simulink library "slib_spectrum_analyser"  (R2020a)
settings: Solver=VariableStepAuto  StartTime=0.0  StopTime=10.0  RelTol=1e-3
libraries: hdlsllib x104, simulink x55, dsphdlxfrm x11, $bdroot x5
(part 2 of 3)

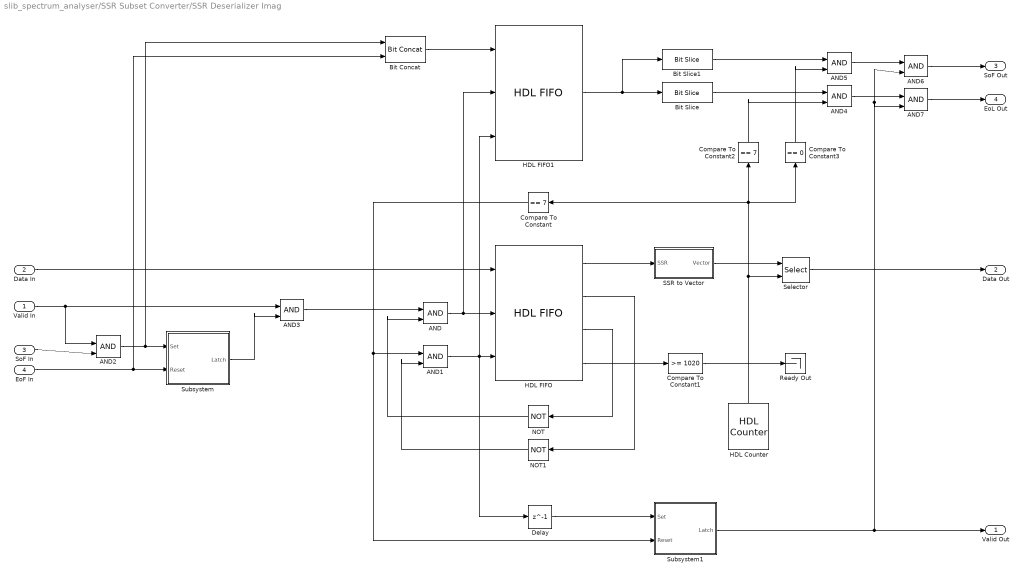
== system slib_spectrum_analyser/SSR Subset Converter/SSR Deserializer Imag ==
  Valid In : Inport
  Data In : Inport  Port=2
  SoF In : Inport  Port=3
  EoF In : Inport  Port=4
  AND{,1..7} (8 alike) : Logic  IconShape=distinctive  AllPortsSameDT=off  OutDataTypeStr=boolean
  Bit Concat : hdlsllib/Logic and Bit Operations/Bit Concat  numInputs=2
  Bit Slice : hdlsllib/Logic and Bit Operations/Bit Slice  lidx=0  ridx=0
      settings: SourceProductBaseCode=SL
  Bit Slice1 : hdlsllib/Logic and Bit Operations/Bit Slice  lidx=1  ridx=1
      settings: SourceProductBaseCode=SL
  Compare To Constant : simulink/Logic and Bit Operations/Compare To Constant  relop===  const=7  OutDataTypeStr=boolean
  Compare To Constant1 : simulink/Logic and Bit Operations/Compare To Constant  relop=>=  const=1020  OutDataTypeStr=boolean
  Compare To Constant2 : simulink/Logic and Bit Operations/Compare To Constant  relop===  const=7  OutDataTypeStr=boolean
  Compare To Constant3 : simulink/Logic and Bit Operations/Compare To Constant  relop===  const=0  OutDataTypeStr=boolean
  Delay : Delay  DelayLength=1
  HDL Counter : hdlsllib/Sources/HDL Counter  CountType=Count limited  CountInit=0  CountStep=1  CountMax=7  CountFromType=Initial value  CountFrom=0  CountResetPort=off  CountLoadPort=off  CountEnbPort=off  CountDirPort=off  CountDataType=Unsigned  CountWordLen=8  CountFracLen=0  CountSampTime=-1
  HDL FIFO : hdlsllib/HDL RAMs/HDL FIFO  fifo_size=1024  mode=Classic  ratio=1  push_msg=Error  pop_msg=Error  show_empty=on  show_full=on  show_num=on  LabelModeActiveChoice_Mode=Classic
      settings: SourceProductBaseCode=SL
  HDL FIFO1 : hdlsllib/HDL RAMs/HDL FIFO  fifo_size=1024  mode=Classic  ratio=1  push_msg=Error  pop_msg=Error  show_empty=off  show_full=off  show_num=off  LabelModeActiveChoice_Mode=Classic
      settings: SourceProductBaseCode=SL
  NOT : Logic  Operator=NOT  IconShape=distinctive  AllPortsSameDT=off  OutDataTypeStr=boolean
  NOT1 : Logic  Operator=NOT  IconShape=distinctive  AllPortsSameDT=off  OutDataTypeStr=boolean
  Ready Out : Terminator
  SSR to Vector : Subsystem  mask{N=8, w=16, hN=8, hw=16}
      mask prompts: N "Samples per clock cycle:"; w "Wordlength:"
      mask init:
      | if ~isequal(get_param(gcb, 'N'), get_param(gcb, 'hN')) ||...
      |         ~isequal(get_param(gcb, 'w'), get_param(gcb, 'hw'))
      |     % Delete all blocks except input and output ports
      |     delete_block(setxor(setdiff(...
      |         find_system(gcb,'LookUnderMasks','on'),...
      |         {[gcb, '/Vector'], [gcb, '/SSR']}), gcb));
      | 
      |     % Delete all wires
      |     delete_line(find_system(gcb, 'FindAll', 'on', 'LookUnderMasks',...
      |         'on', 'SearchDepth', 3, 'Type', 'line', 'Connected', 'off'));
      | 
      |     % Add the matrix concatenation block
      |     add_block('hdlsllib/Math Operations/Matrix Concatenate',...
      |         [gcb, '/Matrix Concatenate'],...
      |         'Position', [155 55 205 330]);
      |     set_param([gcb, '/Matrix Concatenate'], 'NumInputs', num2str(N));
      |     set_param([gcb, '/Matrix Concatenate'], 'Mode', 'Vector');
      |     
      |     % Add wire to output
      |     add_line(gcb, 'Matrix Concatenate/1', 'Vector/1');
      | 
      |     % Add slice blocks and connect wires
      |     for i = 0:N-1
      |         add_block('hdlsllib/Logic and Bit Operations/Bit Slice',...
      |             [gcb, '/Bit Slice', num2str(i)],...
      |             'Position', [0 82+i*90 45 128+i*90]);
      |         set_param([gcb, '/Bit Slice', num2str(i)], 'ridx', num2str(0+i*(w)));
      |         set_param([gcb, '/Bit Slice', num2str(i)], 'lidx', num2str((w-1)+i*(w)));
      |         add_line(gcb, 'SSR/1', ['Bit Slice', num2str(i), '/1'],...
      |             'autorouting', 'on');
      |         add_line(gcb, ['Bit Slice', num2str(i), '/1'],...
      |             ['Matrix Concatenate/', num2str(i+1)],...
      |             'autorouting', 'on');
      |     end
      |     
      |     % Set the hidden attribute to prevent unnecessary changes in
      |     % architecture while generating HDL Code.
      |     set_param(gcb, 'hN', get_param(gcb, 'N'));
      |     set_param(gcb, 'hw', get_param(gcb, 'w'));
      | end
      mask DialogControl DescGroupVar Prompt: SSR to Vector
      mask DialogControl DescTextVar Prompt: Convert the SSR vector format based on the wordlength and expected number of samples per clock cycle.
  Selector : Selector  IndexMode=Zero-based  InputPortWidth=8  IndexOptions=Index vector (port)  Indices=[1 3]  OutputSizes=1
  Subsystem : Subsystem
  Subsystem1 : Subsystem
  Valid Out : Outport
  Data Out : Outport  Port=2
  SoF Out : Outport  Port=3
  EoL Out : Outport  Port=4
  wires:
  Selector/1 -> Data Out/1
  SSR to Vector/1(Vector) -> Selector/1
  Data In/1 -> HDL FIFO/1
  Compare To Constant1/1 -> Ready Out/1
  Compare To Constant3/1 -> AND5/2
  Bit Slice1/1 -> AND5/1
  Bit Slice/1 -> AND4/1
  Compare To Constant2/1 -> AND4/2
  HDL FIFO1/1 -> Bit Slice/1, Bit Slice1/1
  Bit Concat/1 -> HDL FIFO1/1
  Subsystem/1(Latch) -> AND3/2
  HDL FIFO/4 -> Compare To Constant1/1
  Subsystem1/1(Latch) -> AND7/2, AND6/2, Valid Out/1
  NOT1/1 -> AND1/2
  HDL FIFO/2 -> NOT1/1
  Delay/1 -> Subsystem1/1(Set)
  NOT/1 -> AND/2
  EoF In/1 -> Subsystem/2(Reset), Bit Concat/2
  AND3/1 -> AND/1
  Compare To Constant/1 -> AND1/1, Subsystem1/2(Reset)
  AND2/1 -> Subsystem/1(Set), Bit Concat/1
  Valid In/1 -> AND2/1, AND3/1
  SoF In/1 -> AND2/2
  HDL FIFO/3 -> NOT/1
  AND1/1 -> Delay/1, HDL FIFO/3, HDL FIFO1/3
  AND/1 -> HDL FIFO1/2, HDL FIFO/2
  HDL Counter/1 -> Selector/2, Compare To Constant/1, Compare To Constant2/1, Compare To Constant3/1
  HDL FIFO/1 -> SSR to Vector/1(SSR)
  AND5/1 -> AND6/1
  AND6/1 -> SoF Out/1
  AND4/1 -> AND7/1
  AND7/1 -> EoL Out/1

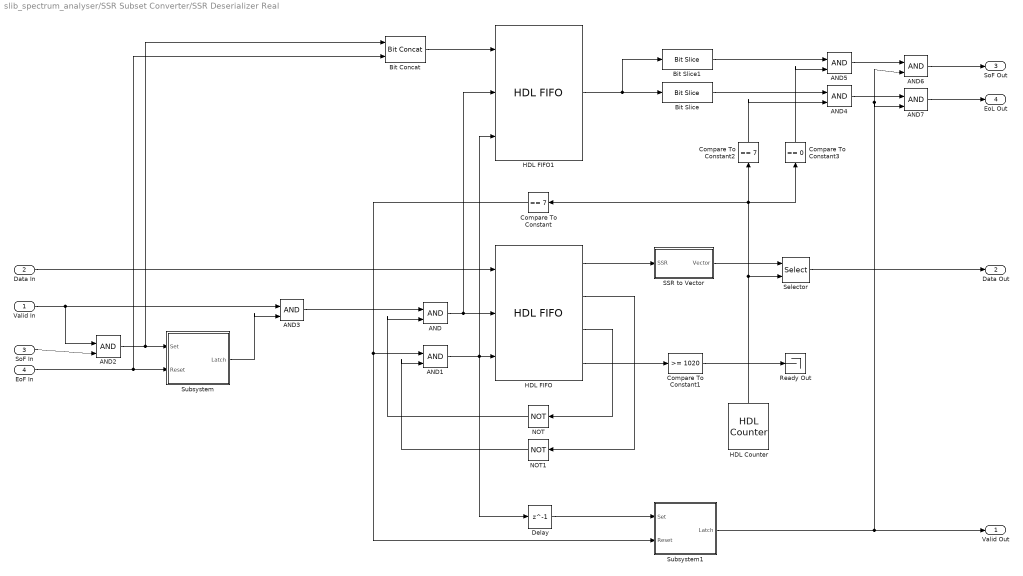
== system slib_spectrum_analyser/SSR Subset Converter/SSR Deserializer Real ==
  Valid In : Inport
  Data In : Inport  Port=2
  SoF In : Inport  Port=3
  EoF In : Inport  Port=4
  AND{,1..7} (8 alike) : Logic  IconShape=distinctive  AllPortsSameDT=off  OutDataTypeStr=boolean
  Bit Concat : hdlsllib/Logic and Bit Operations/Bit Concat  numInputs=2
  Bit Slice : hdlsllib/Logic and Bit Operations/Bit Slice  lidx=0  ridx=0
      settings: SourceProductBaseCode=SL
  Bit Slice1 : hdlsllib/Logic and Bit Operations/Bit Slice  lidx=1  ridx=1
      settings: SourceProductBaseCode=SL
  Compare To Constant : simulink/Logic and Bit Operations/Compare To Constant  relop===  const=7  OutDataTypeStr=boolean
  Compare To Constant1 : simulink/Logic and Bit Operations/Compare To Constant  relop=>=  const=1020  OutDataTypeStr=boolean
  Compare To Constant2 : simulink/Logic and Bit Operations/Compare To Constant  relop===  const=7  OutDataTypeStr=boolean
  Compare To Constant3 : simulink/Logic and Bit Operations/Compare To Constant  relop===  const=0  OutDataTypeStr=boolean
  Delay : Delay  DelayLength=1
  HDL Counter : hdlsllib/Sources/HDL Counter  CountType=Count limited  CountInit=0  CountStep=1  CountMax=7  CountFromType=Initial value  CountFrom=0  CountResetPort=off  CountLoadPort=off  CountEnbPort=off  CountDirPort=off  CountDataType=Unsigned  CountWordLen=8  CountFracLen=0  CountSampTime=-1
  HDL FIFO : hdlsllib/HDL RAMs/HDL FIFO  fifo_size=1024  mode=Classic  ratio=1  push_msg=Error  pop_msg=Error  show_empty=on  show_full=on  show_num=on  LabelModeActiveChoice_Mode=Classic
      settings: SourceProductBaseCode=SL
  HDL FIFO1 : hdlsllib/HDL RAMs/HDL FIFO  fifo_size=1024  mode=Classic  ratio=1  push_msg=Error  pop_msg=Error  show_empty=off  show_full=off  show_num=off  LabelModeActiveChoice_Mode=Classic
      settings: SourceProductBaseCode=SL
  NOT : Logic  Operator=NOT  IconShape=distinctive  AllPortsSameDT=off  OutDataTypeStr=boolean
  NOT1 : Logic  Operator=NOT  IconShape=distinctive  AllPortsSameDT=off  OutDataTypeStr=boolean
  Ready Out : Terminator
  SSR to Vector : Subsystem  mask{N=8, w=16, hN=8, hw=16}
      mask prompts: N "Samples per clock cycle:"; w "Wordlength:"
      mask init: same as slib_spectrum_analyser/SSR Subset Converter/SSR Deserializer Imag/SSR to Vector
      mask DialogControl DescGroupVar Prompt: SSR to Vector
      mask DialogControl DescTextVar Prompt: Convert the SSR vector format based on the wordlength and expected number of samples per clock cycle.
  Selector : Selector  IndexMode=Zero-based  InputPortWidth=8  IndexOptions=Index vector (port)  Indices=[1 3]  OutputSizes=1
  Subsystem : Subsystem
  Subsystem1 : Subsystem
  Valid Out : Outport
  Data Out : Outport  Port=2
  SoF Out : Outport  Port=3
  EoL Out : Outport  Port=4
  wires:
  AND7/1 -> EoL Out/1
  AND4/1 -> AND7/1
  AND6/1 -> SoF Out/1
  AND5/1 -> AND6/1
  HDL FIFO/1 -> SSR to Vector/1(SSR)
  HDL Counter/1 -> Compare To Constant3/1, Compare To Constant2/1, Compare To Constant/1, Selector/2
  AND/1 -> HDL FIFO/2, HDL FIFO1/2
  AND1/1 -> HDL FIFO1/3, HDL FIFO/3, Delay/1
  HDL FIFO/3 -> NOT/1
  SoF In/1 -> AND2/2
  Valid In/1 -> AND3/1, AND2/1
  AND2/1 -> Bit Concat/1, Subsystem/1(Set)
  Compare To Constant/1 -> Subsystem1/2(Reset), AND1/1
  AND3/1 -> AND/1
  EoF In/1 -> Bit Concat/2, Subsystem/2(Reset)
  NOT/1 -> AND/2
  Delay/1 -> Subsystem1/1(Set)
  HDL FIFO/2 -> NOT1/1
  NOT1/1 -> AND1/2
  Subsystem1/1(Latch) -> Valid Out/1, AND6/2, AND7/2
  HDL FIFO/4 -> Compare To Constant1/1
  Subsystem/1(Latch) -> AND3/2
  Bit Concat/1 -> HDL FIFO1/1
  HDL FIFO1/1 -> Bit Slice1/1, Bit Slice/1
  Compare To Constant2/1 -> AND4/2
  Bit Slice/1 -> AND4/1
  Bit Slice1/1 -> AND5/1
  Compare To Constant3/1 -> AND5/2
  Compare To Constant1/1 -> Ready Out/1
  Data In/1 -> HDL FIFO/1
  SSR to Vector/1(Vector) -> Selector/1
  Selector/1 -> Data Out/1

== system slib_spectrum_analyser/SSR Subset Converter/SSR Packet Generator Imag ==
  Frame Drop : Inport
  Valid In : Inport  Port=2
  Data In : Inport  Port=3
  Packet Size : Inport  Port=4
  Frame Dropper : Subsystem
      settings: PortSchema="{\"entries\":[{\"content\":{\"sides\":[{\"content\":{\"connectorIds\":[\"In1\",\"In2\",\"In3\",\"In4\"]},\"type\":\"ConnectorPlacement.EquallySpacedRectSide\",\"uuid\":\"54c30b66-c84f-403b-ae2b-65cc6aec53ae\"},{\"content\":{\"connectorIds\":[\"Out1\",\"Out2\",\"Out3\",\"Out4\"],\"side\":\"RIGHT\"},\"type\":\"ConnectorPlacement.EquallySpacedRectSide\",\"uuid\":\"7fa28ff6-8fce-4ceb-b755-50de3dfb11ba\"},{\"content\":{\"connectorIds\":[\"In5\"],\"side\":\"TOP\"},\"type\":\"ConnectorPlacement.EquallySpacedRectSide\",\"uuid\":\"f3e3849e-6de4-4089-b190-2f6ddd7da8c2\"}]},\"type\":\"ConnectorPlacement.EquallySpacedConnector\",\"uuid\":\"90f0c780-b61a-4293-8926-b92d09c8458c\"}],\"packageUris\":[\"http://schema.mathworks.com/mf0/Connector/19700101\"],\"version\":\"1.0\"}"
  TLAST Generator : Subsystem
  Valid Out : Outport
  Data Out : Outport  Port=2
  SoF Out : Outport  Port=3
  EoF Out : Outport  Port=4
  wires:
  Frame Drop/1 -> Frame Dropper/5(Frame Drop)
  TLAST Generator/4(EoF Out) -> Frame Dropper/4(EoF In)
  TLAST Generator/3(SoF Out) -> Frame Dropper/3(SoF In)
  Frame Dropper/1(Valid Out) -> Valid Out/1
  Frame Dropper/2(Data Out) -> Data Out/1
  Frame Dropper/4(EoF Out) -> EoF Out/1
  Frame Dropper/3(SoF Out) -> SoF Out/1
  TLAST Generator/2(Data Out) -> Frame Dropper/2(Data In)
  TLAST Generator/1(Valid Out) -> Frame Dropper/1(Valid In)
  Packet Size/1 -> TLAST Generator/3(Packet Size)
  Data In/1 -> TLAST Generator/2(Data In)
  Valid In/1 -> TLAST Generator/1(Valid In)

== system slib_spectrum_analyser/SSR Subset Converter/SSR Packet Generator Real ==
  Frame Drop : Inport
  Valid In : Inport  Port=2
  Data In : Inport  Port=3
  Packet Size : Inport  Port=4
  Frame Dropper : Subsystem
      settings: PortSchema="{\"entries\":[{\"content\":{\"sides\":[{\"content\":{\"connectorIds\":[\"In1\",\"In2\",\"In3\",\"In4\"]},\"type\":\"ConnectorPlacement.EquallySpacedRectSide\",\"uuid\":\"54c30b66-c84f-403b-ae2b-65cc6aec53ae\"},{\"content\":{\"connectorIds\":[\"Out1\",\"Out2\",\"Out3\",\"Out4\"],\"side\":\"RIGHT\"},\"type\":\"ConnectorPlacement.EquallySpacedRectSide\",\"uuid\":\"7fa28ff6-8fce-4ceb-b755-50de3dfb11ba\"},{\"content\":{\"connectorIds\":[\"In5\"],\"side\":\"TOP\"},\"type\":\"ConnectorPlacement.EquallySpacedRectSide\",\"uuid\":\"f3e3849e-6de4-4089-b190-2f6ddd7da8c2\"}]},\"type\":\"ConnectorPlacement.EquallySpacedConnector\",\"uuid\":\"90f0c780-b61a-4293-8926-b92d09c8458c\"}],\"packageUris\":[\"http://schema.mathworks.com/mf0/Connector/19700101\"],\"version\":\"1.0\"}"
  TLAST Generator : Subsystem
  Valid Out : Outport
  Data Out : Outport  Port=2
  SoF Out : Outport  Port=3
  EoF Out : Outport  Port=4
  wires:
  Valid In/1 -> TLAST Generator/1(Valid In)
  Data In/1 -> TLAST Generator/2(Data In)
  Packet Size/1 -> TLAST Generator/3(Packet Size)
  TLAST Generator/1(Valid Out) -> Frame Dropper/1(Valid In)
  TLAST Generator/2(Data Out) -> Frame Dropper/2(Data In)
  Frame Dropper/3(SoF Out) -> SoF Out/1
  Frame Dropper/4(EoF Out) -> EoF Out/1
  Frame Dropper/2(Data Out) -> Data Out/1
  Frame Dropper/1(Valid Out) -> Valid Out/1
  TLAST Generator/3(SoF Out) -> Frame Dropper/3(SoF In)
  TLAST Generator/4(EoF Out) -> Frame Dropper/4(EoF In)
  Frame Drop/1 -> Frame Dropper/5(Frame Drop)

== system slib_spectrum_analyser/SSR Subset Converter/SSR Serializer Imag ==
  SSR Control : Inport
  Valid In : Inport  Port=2
  Data In : Inport  Port=3
  Bit Slice : hdlsllib/Logic and Bit Operations/Bit Slice  lidx=0  ridx=0
      settings: SourceProductBaseCode=SL
  Bit Slice1 : hdlsllib/Logic and Bit Operations/Bit Slice  lidx=1  ridx=0
      settings: SourceProductBaseCode=SL
  Delay : Delay  DelayLength=1
  HDL Counter : hdlsllib/Sources/HDL Counter  CountType=Count limited  CountInit=0  CountStep=1  CountMax=7  CountFromType=Initial value  CountFrom=0  CountResetPort=off  CountLoadPort=off  CountEnbPort=on  CountDirPort=off  CountDataType=Unsigned  CountWordLen=3  CountFracLen=0  CountSampTime=1
  Multiport Switch : MultiPortSwitch  DataPortOrder=Zero-based contiguous  Inputs=4  zeroidx=on
  Multiport Switch1 : MultiPortSwitch  DataPortOrder=Zero-based contiguous  Inputs=4  zeroidx=on
  SSR to Vector : Subsystem  mask{N=8, w=16, hN=8, hw=16}
      mask prompts: N "Samples per clock cycle:"; w "Wordlength:"
      mask init: same as slib_spectrum_analyser/SSR Subset Converter/SSR Deserializer Imag/SSR to Vector
      mask DialogControl DescGroupVar Prompt: SSR to Vector
      mask DialogControl DescTextVar Prompt: Convert the SSR vector format based on the wordlength and expected number of samples per clock cycle.
  SSR1 to SSR8 : Subsystem
  SSR2 to SSR8 : Subsystem
  SSR4 to SSR8 : Subsystem
  Unit Delay Enabled Synchronous : hdlsllib/Discrete/Unit Delay Enabled Synchronous  InitialCondition=0.0  SampleTime=-1
      settings: SourceProductBaseCode=SL
  Vector to SSR : Subsystem  mask{N=8, hN=8}
      mask prompts: N "Samples per clock cycle:"
      mask init:
      | if ~isequal(get_param(gcb, 'N'), get_param(gcb, 'hN'))
      |     % Delete all blocks except input and output ports
      |     delete_block(setxor(setdiff(...
      |         find_system(gcb,'LookUnderMasks','on'),...
      |         {[gcb, '/Vector'], [gcb, '/SSR']}), gcb));
      | 
      |     % Delete all wires
      |     delete_line(find_system(gcb, 'FindAll', 'on', 'LookUnderMasks',...
      |         'on', 'SearchDepth', 3, 'Type', 'line', 'Connected', 'off'));
      | 
      |     % Add the bit concatenation block
      |     add_block('hdlsllib/Logic and Bit Operations/Bit Concat',...
      |         [gcb, '/Bit Concat'],...
      |         'Position', [155 55 205 330]);
      |     set_param([gcb, '/Bit Concat'], 'numInputs', num2str(N));
      | 
      |     % Add wire to output
      |     add_line(gcb, 'Bit Concat/1', 'SSR/1');
      | 
      |     % Add selector blocks and connect wires
      |     for i = 0:N-1
      |         add_block('simulink/Signal Routing/Selector',...
      |             [gcb, '/Selector', num2str(i)],...
      |             'Position', [0 82+i*90 45 128+i*90]);
      |         set_param([gcb, '/Selector', num2str(i)], 'InputPortWidth', num2str(N));
      |         set_param([gcb, '/Selector', num2str(i)], 'IndexParamArray', {num2str(N-i)});
      |         add_line(gcb, 'Vector/1', ['Selector', num2str(i), '/1'],...
      |             'autorouting', 'on');
      |         add_line(gcb, ['Selector', num2str(i), '/1'],...
      |             ['Bit Concat/', num2str(i+1)],...
      |             'autorouting', 'on');
      |     end
      |     
      |     % Set the hidden attribute to prevent unnecessary changes in
      |     % architecture while generating HDL Code.
      |     set_param(gcb, 'hN', get_param(gcb, 'N'));
      | end
      mask DialogControl DescGroupVar Prompt: Vector to SSR
      mask DialogControl DescTextVar Prompt: Convert a vector of inputs into SSR format.
  Valid Out : Outport
  Data Out : Outport  Port=2
  wires:
  Vector to SSR/1(SSR) -> Data Out/1
  SSR to Vector/1(Vector) -> SSR4 to SSR8/1(Data In), SSR2 to SSR8/1(Data In), SSR1 to SSR8/1(Data In), Multiport Switch/5
  Unit Delay Enabled Synchronous/1 -> Vector to SSR/1(Vector)
  Multiport Switch/1 -> Unit Delay Enabled Synchronous/1
  Delay/1 -> Valid Out/1
  Valid In/1 -> SSR2 to SSR8/3(Valid In), SSR1 to SSR8/3(Valid In), HDL Counter/1, Multiport Switch1/5, SSR4 to SSR8/3(Valid In)
  SSR4 to SSR8/2(Valid Out) -> Multiport Switch1/4
  SSR2 to SSR8/2(Valid Out) -> Multiport Switch1/3
  SSR1 to SSR8/2(Valid Out) -> Multiport Switch1/2
  Bit Slice/1 -> SSR4 to SSR8/2(Index)
  SSR Control/1 -> Multiport Switch/1, Multiport Switch1/1
  HDL Counter/1 -> SSR1 to SSR8/2(Index), Bit Slice1/1, Bit Slice/1
  Bit Slice1/1 -> SSR2 to SSR8/2(Index)
  Data In/1 -> SSR to Vector/1(SSR)
  SSR1 to SSR8/1(Data Out) -> Multiport Switch/2
  SSR2 to SSR8/1(Data Out) -> Multiport Switch/3
  SSR4 to SSR8/1(Data Out) -> Multiport Switch/4
  Multiport Switch1/1 -> Unit Delay Enabled Synchronous/2, Delay/1

== system slib_spectrum_analyser/SSR Subset Converter/SSR Serializer Real ==
  SSR Control : Inport
  Valid In : Inport  Port=2
  Data In : Inport  Port=3
  Bit Slice : hdlsllib/Logic and Bit Operations/Bit Slice  lidx=0  ridx=0
      settings: SourceProductBaseCode=SL
  Bit Slice1 : hdlsllib/Logic and Bit Operations/Bit Slice  lidx=1  ridx=0
      settings: SourceProductBaseCode=SL
  Delay : Delay  DelayLength=1
  HDL Counter : hdlsllib/Sources/HDL Counter  CountType=Count limited  CountInit=0  CountStep=1  CountMax=7  CountFromType=Initial value  CountFrom=0  CountResetPort=off  CountLoadPort=off  CountEnbPort=on  CountDirPort=off  CountDataType=Unsigned  CountWordLen=3  CountFracLen=0  CountSampTime=1
  Multiport Switch : MultiPortSwitch  DataPortOrder=Zero-based contiguous  Inputs=4  zeroidx=on
  Multiport Switch1 : MultiPortSwitch  DataPortOrder=Zero-based contiguous  Inputs=4  zeroidx=on
  SSR to Vector : Subsystem  mask{N=8, w=16, hN=8, hw=16}
      mask prompts: N "Samples per clock cycle:"; w "Wordlength:"
      mask init: same as slib_spectrum_analyser/SSR Subset Converter/SSR Deserializer Imag/SSR to Vector
      mask DialogControl DescGroupVar Prompt: SSR to Vector
      mask DialogControl DescTextVar Prompt: Convert the SSR vector format based on the wordlength and expected number of samples per clock cycle.
  SSR1 to SSR8 : Subsystem
  SSR2 to SSR8 : Subsystem
  SSR4 to SSR8 : Subsystem
  Unit Delay Enabled Synchronous : hdlsllib/Discrete/Unit Delay Enabled Synchronous  InitialCondition=0.0  SampleTime=-1
      settings: SourceProductBaseCode=SL
  Vector to SSR : Subsystem  mask{N=8, hN=8}
      mask prompts: N "Samples per clock cycle:"
      mask init: same as slib_spectrum_analyser/SSR Subset Converter/SSR Serializer Imag/Vector to SSR
      mask DialogControl DescGroupVar Prompt: Vector to SSR
      mask DialogControl DescTextVar Prompt: Convert a vector of inputs into SSR format.
  Valid Out : Outport
  Data Out : Outport  Port=2
  wires:
  Multiport Switch1/1 -> Delay/1, Unit Delay Enabled Synchronous/2
  SSR4 to SSR8/1(Data Out) -> Multiport Switch/4
  SSR2 to SSR8/1(Data Out) -> Multiport Switch/3
  SSR1 to SSR8/1(Data Out) -> Multiport Switch/2
  Data In/1 -> SSR to Vector/1(SSR)
  Bit Slice1/1 -> SSR2 to SSR8/2(Index)
  HDL Counter/1 -> Bit Slice/1, Bit Slice1/1, SSR1 to SSR8/2(Index)
  SSR Control/1 -> Multiport Switch1/1, Multiport Switch/1
  Bit Slice/1 -> SSR4 to SSR8/2(Index)
  SSR1 to SSR8/2(Valid Out) -> Multiport Switch1/2
  SSR2 to SSR8/2(Valid Out) -> Multiport Switch1/3
  SSR4 to SSR8/2(Valid Out) -> Multiport Switch1/4
  Valid In/1 -> SSR4 to SSR8/3(Valid In), Multiport Switch1/5, HDL Counter/1, SSR1 to SSR8/3(Valid In), SSR2 to SSR8/3(Valid In)
  Delay/1 -> Valid Out/1
  Multiport Switch/1 -> Unit Delay Enabled Synchronous/1
  Unit Delay Enabled Synchronous/1 -> Vector to SSR/1(Vector)
  SSR to Vector/1(Vector) -> Multiport Switch/5, SSR1 to SSR8/1(Data In), SSR2 to SSR8/1(Data In), SSR4 to SSR8/1(Data In)
  Vector to SSR/1(SSR) -> Data Out/1

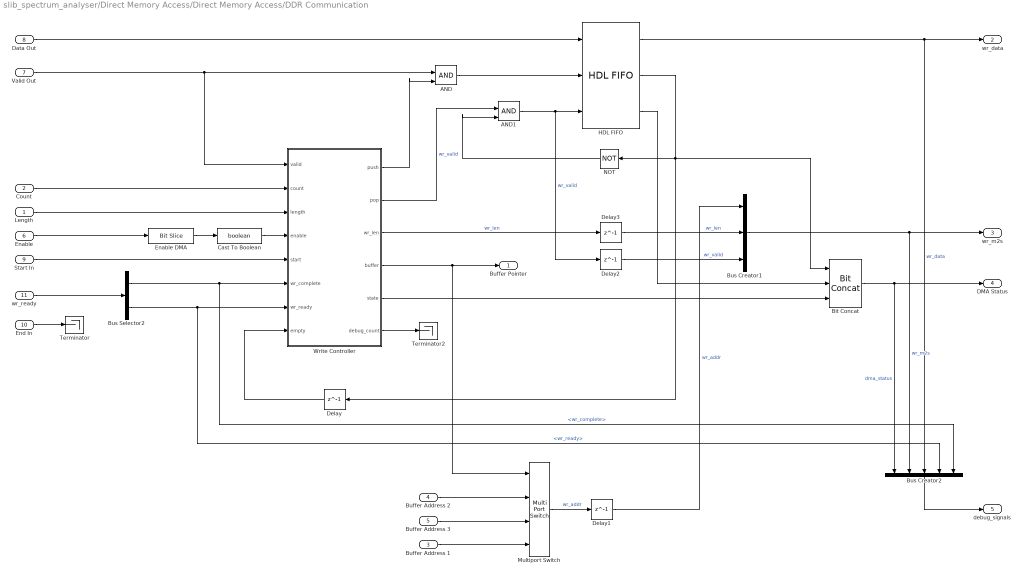
== system slib_spectrum_analyser/Direct Memory Access/Direct Memory Access/DDR Communication ==
  Length : Inport
  Count : Inport  Port=2
  Buffer Address 1 : Inport  Port=3
  Buffer Address 2 : Inport  Port=4
  Buffer Address 3 : Inport  Port=5
  Enable : Inport  Port=6
  Valid Out : Inport  Port=7
  Data Out : Inport  Port=8
  Start In : Inport  Port=9
  End In : Inport  Port=10
  wr_ready : Inport  Port=11
  AND : Logic  IconShape=distinctive  AllPortsSameDT=off  OutDataTypeStr=boolean
  AND1 : Logic  IconShape=distinctive  AllPortsSameDT=off  OutDataTypeStr=boolean
  Bit Concat : hdlsllib/Logic and Bit Operations/Bit Concat  numInputs=3
  Bus Creator1 : BusCreator  Inputs=3
  Bus Creator2 : BusCreator  Inputs=5
  Bus Selector2 : BusSelector  OutputSignals=wr_complete,wr_ready
  Cast To Boolean : DataTypeConversion  OutDataTypeStr=boolean
  Delay{,1..3} (4 alike) : Delay  DelayLength=1
  Enable DMA : hdlsllib/Logic and Bit Operations/Bit Slice  lidx=0  ridx=0
      settings: SourceProductBaseCode=SL
  HDL FIFO : hdlsllib/HDL RAMs/HDL FIFO  fifo_size=8192  mode=Classic  ratio=1  push_msg=Error  pop_msg=Error  show_empty=on  show_full=on  show_num=off  LabelModeActiveChoice_Mode=Classic
      settings: SourceProductBaseCode=SL
  Multiport Switch : MultiPortSwitch  DataPortOrder=Zero-based contiguous  zeroidx=on
  NOT : Logic  Operator=NOT  IconShape=distinctive  AllPortsSameDT=off  OutDataTypeStr=boolean
  Terminator : Terminator
  Terminator2 : Terminator
  Write Controller : MATLAB Function  TreatAsAtomicUnit=on
  Buffer Pointer : Outport
  wr_data : Outport  Port=2
  wr_m2s : Outport  Port=3  VectorParamsAs1DForOutWhenUnconnected=off
  DMA Status : Outport  Port=4
  debug_signals : Outport  Port=5
  wires:
  Buffer Address 3/1 -> Multiport Switch/3
  Buffer Address 2/1 -> Multiport Switch/2
  Buffer Address 1/1 -> Multiport Switch/4
  Multiport Switch/1 -> Delay1/1  "wr_addr"
  Delay/1 -> Write Controller/8(empty)
  Data Out/1 -> HDL FIFO/1
  NOT/1 -> AND1/2
  AND1/1 -> Delay2/1, HDL FIFO/3  "wr_valid"
  wr_ready/1 -> Bus Selector2/1
  Bus Creator1/1 -> Bus Creator2/2, wr_m2s/1  "wr_m2s"
  Write Controller/1(push) -> AND/2
  HDL FIFO/1 -> Bus Creator2/3, wr_data/1  "wr_data"
  Valid Out/1 -> Write Controller/1(valid), AND/1
  AND/1 -> HDL FIFO/2
  HDL FIFO/2 -> Delay/1, Bit Concat/1, NOT/1
  Enable/1 -> Enable DMA/1
  End In/1 -> Terminator/1
  Write Controller/4(buffer) -> Buffer Pointer/1, Multiport Switch/1
  Bit Concat/1 -> Bus Creator2/1, DMA Status/1  "dma_status"
  Write Controller/5(state) -> Bit Concat/3
  HDL FIFO/3 -> Bit Concat/2
  Length/1 -> Write Controller/3(length)
  Write Controller/6(debug_count) -> Terminator2/1
  Start In/1 -> Write Controller/5(start)
  Write Controller/2(pop) -> AND1/1  "wr_valid"
  Bus Selector2/2 -> Write Controller/7(wr_ready), Bus Creator2/4  "<wr_ready>"
  Enable DMA/1 -> Cast To Boolean/1
  Cast To Boolean/1 -> Write Controller/4(enable)
  Bus Creator2/1 -> debug_signals/1
  Count/1 -> Write Controller/2(count)
  Bus Selector2/1 -> Bus Creator2/5, Write Controller/6(wr_complete)  "<wr_complete>"
  Write Controller/3(wr_len) -> Delay3/1  "wr_len"
  Delay1/1 -> Bus Creator1/1  "wr_addr"
  Delay2/1 -> Bus Creator1/3  "wr_valid"
  Delay3/1 -> Bus Creator1/2  "wr_len"

== system slib_spectrum_analyser/Preprocessing Window/Direct Memory Access/EdgeDetection ==
  In1 : Inport
  Delay : Delay  DelayLength=1
  Logical Operator : Logic  AllPortsSameDT=off  OutDataTypeStr=boolean
  Logical Operator1 : Logic  Operator=NOT  AllPortsSameDT=off  OutDataTypeStr=boolean
  Out1 : Outport  VectorParamsAs1DForOutWhenUnconnected=off
  wires:
  Logical Operator/1 -> Out1/1
  Logical Operator1/1 -> Logical Operator/1
  Delay/1 -> Logical Operator1/1
  In1/1 -> Delay/1, Logical Operator/2

== system slib_spectrum_analyser/SSR Subset Converter/SSR Deserializer Imag/SSR to Vector ==
  SSR : Inport
  Bit Slice0 : hdlsllib/Logic and Bit Operations/Bit Slice  lidx=15  ridx=0
      settings: SourceProductBaseCode=SL
  Bit Slice1 : hdlsllib/Logic and Bit Operations/Bit Slice  lidx=31  ridx=16
      settings: SourceProductBaseCode=SL
  Bit Slice2 : hdlsllib/Logic and Bit Operations/Bit Slice  lidx=47  ridx=32
      settings: SourceProductBaseCode=SL
  Bit Slice3 : hdlsllib/Logic and Bit Operations/Bit Slice  lidx=63  ridx=48
      settings: SourceProductBaseCode=SL
  Bit Slice4 : hdlsllib/Logic and Bit Operations/Bit Slice  lidx=79  ridx=64
      settings: SourceProductBaseCode=SL
  Bit Slice5 : hdlsllib/Logic and Bit Operations/Bit Slice  lidx=95  ridx=80
      settings: SourceProductBaseCode=SL
  Bit Slice6 : hdlsllib/Logic and Bit Operations/Bit Slice  lidx=111  ridx=96
      settings: SourceProductBaseCode=SL
  Bit Slice7 : hdlsllib/Logic and Bit Operations/Bit Slice  lidx=127  ridx=112
      settings: SourceProductBaseCode=SL
  Matrix Concatenate : Concatenate  NumInputs=8  ConcatenateDimension=2
  Vector : Outport
  wires:
  Bit Slice7/1 -> Matrix Concatenate/8
  Bit Slice6/1 -> Matrix Concatenate/7
  Bit Slice5/1 -> Matrix Concatenate/6
  Bit Slice4/1 -> Matrix Concatenate/5
  Bit Slice3/1 -> Matrix Concatenate/4
  Bit Slice2/1 -> Matrix Concatenate/3
  Bit Slice1/1 -> Matrix Concatenate/2
  Bit Slice0/1 -> Matrix Concatenate/1
  SSR/1 -> Bit Slice0/1, Bit Slice1/1, Bit Slice2/1, Bit Slice3/1, Bit Slice4/1, Bit Slice5/1, Bit Slice7/1, Bit Slice6/1
  Matrix Concatenate/1 -> Vector/1

== system slib_spectrum_analyser/SSR Subset Converter/SSR Deserializer Imag/Subsystem ==
  Set : Inport
  Reset : Inport  Port=2
  Constant : Constant  OutDataTypeStr=boolean  SampleTime=-1
  Multiport Switch : MultiPortSwitch  DataPortOrder=Zero-based contiguous  Inputs=2  zeroidx=on
  Unit Delay Resettable Synchronous : hdlsllib/Discrete/Unit Delay Resettable Synchronous  InitialCondition=0.0  SampleTime=-1
      settings: SourceProductBaseCode=SL
  Latch : Outport
  wires:
  Multiport Switch/1 -> Unit Delay Resettable Synchronous/1, Latch/1
  Set/1 -> Multiport Switch/1
  Reset/1 -> Unit Delay Resettable Synchronous/2
  Constant/1 -> Multiport Switch/3
  Unit Delay Resettable Synchronous/1 -> Multiport Switch/2

== system slib_spectrum_analyser/SSR Subset Converter/SSR Deserializer Imag/Subsystem1 ==
  Set : Inport
  Reset : Inport  Port=2
  Constant : Constant  OutDataTypeStr=boolean  SampleTime=-1
  Multiport Switch : MultiPortSwitch  DataPortOrder=Zero-based contiguous  Inputs=2  zeroidx=on
  Unit Delay Resettable Synchronous : hdlsllib/Discrete/Unit Delay Resettable Synchronous  InitialCondition=0.0  SampleTime=-1
      settings: SourceProductBaseCode=SL
  Latch : Outport
  wires:
  Unit Delay Resettable Synchronous/1 -> Multiport Switch/2
  Constant/1 -> Multiport Switch/3
  Reset/1 -> Unit Delay Resettable Synchronous/2
  Set/1 -> Multiport Switch/1
  Multiport Switch/1 -> Latch/1, Unit Delay Resettable Synchronous/1

== system slib_spectrum_analyser/SSR Subset Converter/SSR Deserializer Real/SSR to Vector ==
  SSR : Inport
  Bit Slice0 : hdlsllib/Logic and Bit Operations/Bit Slice  lidx=15  ridx=0
      settings: SourceProductBaseCode=SL
  Bit Slice1 : hdlsllib/Logic and Bit Operations/Bit Slice  lidx=31  ridx=16
      settings: SourceProductBaseCode=SL
  Bit Slice2 : hdlsllib/Logic and Bit Operations/Bit Slice  lidx=47  ridx=32
      settings: SourceProductBaseCode=SL
  Bit Slice3 : hdlsllib/Logic and Bit Operations/Bit Slice  lidx=63  ridx=48
      settings: SourceProductBaseCode=SL
  Bit Slice4 : hdlsllib/Logic and Bit Operations/Bit Slice  lidx=79  ridx=64
      settings: SourceProductBaseCode=SL
  Bit Slice5 : hdlsllib/Logic and Bit Operations/Bit Slice  lidx=95  ridx=80
      settings: SourceProductBaseCode=SL
  Bit Slice6 : hdlsllib/Logic and Bit Operations/Bit Slice  lidx=111  ridx=96
      settings: SourceProductBaseCode=SL
  Bit Slice7 : hdlsllib/Logic and Bit Operations/Bit Slice  lidx=127  ridx=112
      settings: SourceProductBaseCode=SL
  Matrix Concatenate : Concatenate  NumInputs=8  ConcatenateDimension=2
  Vector : Outport
  wires:
  Matrix Concatenate/1 -> Vector/1
  SSR/1 -> Bit Slice6/1, Bit Slice7/1, Bit Slice5/1, Bit Slice4/1, Bit Slice3/1, Bit Slice2/1, Bit Slice1/1, Bit Slice0/1
  Bit Slice0/1 -> Matrix Concatenate/1
  Bit Slice1/1 -> Matrix Concatenate/2
  Bit Slice2/1 -> Matrix Concatenate/3
  Bit Slice3/1 -> Matrix Concatenate/4
  Bit Slice4/1 -> Matrix Concatenate/5
  Bit Slice5/1 -> Matrix Concatenate/6
  Bit Slice6/1 -> Matrix Concatenate/7
  Bit Slice7/1 -> Matrix Concatenate/8

== system slib_spectrum_analyser/SSR Subset Converter/SSR Deserializer Real/Subsystem ==
  Set : Inport
  Reset : Inport  Port=2
  Constant : Constant  OutDataTypeStr=boolean  SampleTime=-1
  Multiport Switch : MultiPortSwitch  DataPortOrder=Zero-based contiguous  Inputs=2  zeroidx=on
  Unit Delay Resettable Synchronous : hdlsllib/Discrete/Unit Delay Resettable Synchronous  InitialCondition=0.0  SampleTime=-1
      settings: SourceProductBaseCode=SL
  Latch : Outport
  wires:
  Unit Delay Resettable Synchronous/1 -> Multiport Switch/2
  Constant/1 -> Multiport Switch/3
  Reset/1 -> Unit Delay Resettable Synchronous/2
  Set/1 -> Multiport Switch/1
  Multiport Switch/1 -> Latch/1, Unit Delay Resettable Synchronous/1

== system slib_spectrum_analyser/SSR Subset Converter/SSR Deserializer Real/Subsystem1 ==
  Set : Inport
  Reset : Inport  Port=2
  Constant : Constant  OutDataTypeStr=boolean  SampleTime=-1
  Multiport Switch : MultiPortSwitch  DataPortOrder=Zero-based contiguous  Inputs=2  zeroidx=on
  Unit Delay Resettable Synchronous : hdlsllib/Discrete/Unit Delay Resettable Synchronous  InitialCondition=0.0  SampleTime=-1
      settings: SourceProductBaseCode=SL
  Latch : Outport
  wires:
  Multiport Switch/1 -> Unit Delay Resettable Synchronous/1, Latch/1
  Set/1 -> Multiport Switch/1
  Reset/1 -> Unit Delay Resettable Synchronous/2
  Constant/1 -> Multiport Switch/3
  Unit Delay Resettable Synchronous/1 -> Multiport Switch/2

== system slib_spectrum_analyser/SSR Subset Converter/SSR Packet Generator Imag/Frame Dropper ==
  Valid In : Inport
  Data In : Inport  Port=2
  SoF In : Inport  Port=3
  EoF In : Inport  Port=4
  Frame Drop : Inport  Port=5
  AND : Logic  IconShape=distinctive  AllPortsSameDT=off  OutDataTypeStr=boolean
  AND1 : Logic  IconShape=distinctive  AllPortsSameDT=off  OutDataTypeStr=boolean
  AND2 : Logic  IconShape=distinctive  AllPortsSameDT=off  OutDataTypeStr=boolean
  Compare To Zero : simulink/Logic and Bit Operations/Compare To Zero  relop===  OutDataTypeStr=boolean
  Constant : Constant  Value=0  OutDataTypeStr=fixdt(0,4,0)  SampleTime=-1
  Constant1 : Constant  OutDataTypeStr=fixdt(0,4,0)  SampleTime=-1
  HDL Counter : hdlsllib/Sources/HDL Counter  CountType=Count limited  CountInit=0  CountStep=1  CountMax=7  CountFromType=Initial value  CountFrom=0  CountResetPort=on  CountLoadPort=off  CountEnbPort=on  CountDirPort=off  CountDataType=Unsigned  CountWordLen=4  CountFracLen=0  CountSampTime=1
  Multiport Switch : MultiPortSwitch  DataPortOrder=Zero-based contiguous  Inputs=2  zeroidx=on
  Relational Operator : RelationalOperator  Operator=<=  OutDataTypeStr=boolean  RndMeth=Simplest
  Shift Arithmetic : ArithShift  BitShiftNumberSource=Input port  BitShiftNumber=8  BitShiftDirection=Left
      settings: InputPortMap=u0,p1
  Valid Out : Outport
  Data Out : Outport  Port=2
  SoF Out : Outport  Port=3
  EoF Out : Outport  Port=4
  wires:
  Constant1/1 -> Shift Arithmetic/1
  Frame Drop/1 -> Shift Arithmetic/2
  Shift Arithmetic/1 -> Relational Operator/1
  HDL Counter/1 -> Multiport Switch/2, Relational Operator/2
  Constant/1 -> Multiport Switch/3
  Multiport Switch/1 -> Compare To Zero/1
  Relational Operator/1 -> Multiport Switch/1, HDL Counter/1
  SoF In/1 -> AND2/2
  AND2/1 -> SoF Out/1
  AND1/1 -> EoF Out/1
  EoF In/1 -> HDL Counter/2, AND1/2
  AND/1 -> Valid Out/1
  Compare To Zero/1 -> AND1/1, AND2/1, AND/2
  Valid In/1 -> AND/1
  Data In/1 -> Data Out/1

== system slib_spectrum_analyser/SSR Subset Converter/SSR Packet Generator Imag/TLAST Generator ==
  Valid In : Inport
  Data In : Inport  Port=2
  Packet Size : Inport  Port=3
  AND : Logic  Inputs=3  IconShape=distinctive  AllPortsSameDT=off  OutDataTypeStr=boolean
  AND1 : Logic  Inputs=3  IconShape=distinctive  AllPortsSameDT=off  OutDataTypeStr=boolean
  AND2 : Logic  IconShape=distinctive  AllPortsSameDT=off  OutDataTypeStr=boolean
  AND3 : Logic  IconShape=distinctive  AllPortsSameDT=off  OutDataTypeStr=boolean
  Compare To Constant : simulink/Logic and Bit Operations/Compare To Constant  relop===  const=1  OutDataTypeStr=boolean
  Compare To Zero : simulink/Logic and Bit Operations/Compare To Zero  relop=~=  OutDataTypeStr=boolean
  HDL Counter : hdlsllib/Sources/HDL Counter  CountType=Free running  CountInit=1  CountStep=1  CountMax=7  CountFromType=Initial value  CountFrom=1  CountResetPort=on  CountLoadPort=off  CountEnbPort=on  CountDirPort=off  CountDataType=Unsigned  CountWordLen=32  CountFracLen=0  CountSampTime=1
  Relational Operator : RelationalOperator  Operator=<=  OutDataTypeStr=boolean  RndMeth=Simplest
  Unit Delay Enabled Synchronous : hdlsllib/Discrete/Unit Delay Enabled Synchronous  InitialCondition=0.0  SampleTime=-1
      settings: SourceProductBaseCode=SL
  Valid Out : Outport
  Data Out : Outport  Port=2
  SoF Out : Outport  Port=3
  EoF Out : Outport  Port=4
  wires:
  AND/1 -> SoF Out/1
  Compare To Constant/1 -> AND/1
  Data In/1 -> Data Out/1
  AND1/1 -> HDL Counter/1, EoF Out/1
  Compare To Zero/1 -> AND1/3, AND/3, AND2/1
  AND2/1 -> Valid Out/1
  HDL Counter/1 -> Relational Operator/2, Compare To Constant/1
  Packet Size/1 -> Unit Delay Enabled Synchronous/1
  Unit Delay Enabled Synchronous/1 -> Compare To Zero/1, Relational Operator/1
  Relational Operator/1 -> AND3/2, AND1/1
  Valid In/1 -> AND3/1, AND1/2, AND/2, AND2/2, HDL Counter/2
  AND3/1 -> Unit Delay Enabled Synchronous/2

== system slib_spectrum_analyser/SSR Subset Converter/SSR Packet Generator Real/Frame Dropper ==
  Valid In : Inport
  Data In : Inport  Port=2
  SoF In : Inport  Port=3
  EoF In : Inport  Port=4
  Frame Drop : Inport  Port=5
  AND : Logic  IconShape=distinctive  AllPortsSameDT=off  OutDataTypeStr=boolean
  AND1 : Logic  IconShape=distinctive  AllPortsSameDT=off  OutDataTypeStr=boolean
  AND2 : Logic  IconShape=distinctive  AllPortsSameDT=off  OutDataTypeStr=boolean
  Compare To Zero : simulink/Logic and Bit Operations/Compare To Zero  relop===  OutDataTypeStr=boolean
  Constant : Constant  Value=0  OutDataTypeStr=fixdt(0,4,0)  SampleTime=-1
  Constant1 : Constant  OutDataTypeStr=fixdt(0,4,0)  SampleTime=-1
  HDL Counter : hdlsllib/Sources/HDL Counter  CountType=Count limited  CountInit=0  CountStep=1  CountMax=7  CountFromType=Initial value  CountFrom=0  CountResetPort=on  CountLoadPort=off  CountEnbPort=on  CountDirPort=off  CountDataType=Unsigned  CountWordLen=4  CountFracLen=0  CountSampTime=1
  Multiport Switch : MultiPortSwitch  DataPortOrder=Zero-based contiguous  Inputs=2  zeroidx=on
  Relational Operator : RelationalOperator  Operator=<=  OutDataTypeStr=boolean  RndMeth=Simplest
  Shift Arithmetic : ArithShift  BitShiftNumberSource=Input port  BitShiftNumber=8  BitShiftDirection=Left
      settings: InputPortMap=u0,p1
  Valid Out : Outport
  Data Out : Outport  Port=2
  SoF Out : Outport  Port=3
  EoF Out : Outport  Port=4
  wires:
  Data In/1 -> Data Out/1
  Valid In/1 -> AND/1
  Compare To Zero/1 -> AND/2, AND2/1, AND1/1
  AND/1 -> Valid Out/1
  EoF In/1 -> AND1/2, HDL Counter/2
  AND1/1 -> EoF Out/1
  AND2/1 -> SoF Out/1
  SoF In/1 -> AND2/2
  Relational Operator/1 -> HDL Counter/1, Multiport Switch/1
  Multiport Switch/1 -> Compare To Zero/1
  Constant/1 -> Multiport Switch/3
  HDL Counter/1 -> Relational Operator/2, Multiport Switch/2
  Shift Arithmetic/1 -> Relational Operator/1
  Frame Drop/1 -> Shift Arithmetic/2
  Constant1/1 -> Shift Arithmetic/1

== system slib_spectrum_analyser/SSR Subset Converter/SSR Packet Generator Real/TLAST Generator ==
  Valid In : Inport
  Data In : Inport  Port=2
  Packet Size : Inport  Port=3
  AND : Logic  Inputs=3  IconShape=distinctive  AllPortsSameDT=off  OutDataTypeStr=boolean
  AND1 : Logic  Inputs=3  IconShape=distinctive  AllPortsSameDT=off  OutDataTypeStr=boolean
  AND2 : Logic  IconShape=distinctive  AllPortsSameDT=off  OutDataTypeStr=boolean
  AND3 : Logic  IconShape=distinctive  AllPortsSameDT=off  OutDataTypeStr=boolean
  Compare To Constant : simulink/Logic and Bit Operations/Compare To Constant  relop===  const=1  OutDataTypeStr=boolean
  Compare To Zero : simulink/Logic and Bit Operations/Compare To Zero  relop=~=  OutDataTypeStr=boolean
  HDL Counter : hdlsllib/Sources/HDL Counter  CountType=Free running  CountInit=1  CountStep=1  CountMax=7  CountFromType=Initial value  CountFrom=1  CountResetPort=on  CountLoadPort=off  CountEnbPort=on  CountDirPort=off  CountDataType=Unsigned  CountWordLen=32  CountFracLen=0  CountSampTime=1
  Relational Operator : RelationalOperator  Operator=<=  OutDataTypeStr=boolean  RndMeth=Simplest
  Unit Delay Enabled Synchronous : hdlsllib/Discrete/Unit Delay Enabled Synchronous  InitialCondition=0.0  SampleTime=-1
      settings: SourceProductBaseCode=SL
  Valid Out : Outport
  Data Out : Outport  Port=2
  SoF Out : Outport  Port=3
  EoF Out : Outport  Port=4
  wires:
  AND3/1 -> Unit Delay Enabled Synchronous/2
  Valid In/1 -> HDL Counter/2, AND2/2, AND/2, AND1/2, AND3/1
  Relational Operator/1 -> AND1/1, AND3/2
  Unit Delay Enabled Synchronous/1 -> Relational Operator/1, Compare To Zero/1
  Packet Size/1 -> Unit Delay Enabled Synchronous/1
  HDL Counter/1 -> Compare To Constant/1, Relational Operator/2
  AND2/1 -> Valid Out/1
  Compare To Zero/1 -> AND2/1, AND/3, AND1/3
  AND1/1 -> EoF Out/1, HDL Counter/1
  Data In/1 -> Data Out/1
  Compare To Constant/1 -> AND/1
  AND/1 -> SoF Out/1

== system slib_spectrum_analyser/SSR Subset Converter/SSR Serializer Imag/SSR to Vector ==
  SSR : Inport
  Bit Slice0 : hdlsllib/Logic and Bit Operations/Bit Slice  lidx=15  ridx=0
      settings: SourceProductBaseCode=SL
  Bit Slice1 : hdlsllib/Logic and Bit Operations/Bit Slice  lidx=31  ridx=16
      settings: SourceProductBaseCode=SL
  Bit Slice2 : hdlsllib/Logic and Bit Operations/Bit Slice  lidx=47  ridx=32
      settings: SourceProductBaseCode=SL
  Bit Slice3 : hdlsllib/Logic and Bit Operations/Bit Slice  lidx=63  ridx=48
      settings: SourceProductBaseCode=SL
  Bit Slice4 : hdlsllib/Logic and Bit Operations/Bit Slice  lidx=79  ridx=64
      settings: SourceProductBaseCode=SL
  Bit Slice5 : hdlsllib/Logic and Bit Operations/Bit Slice  lidx=95  ridx=80
      settings: SourceProductBaseCode=SL
  Bit Slice6 : hdlsllib/Logic and Bit Operations/Bit Slice  lidx=111  ridx=96
      settings: SourceProductBaseCode=SL
  Bit Slice7 : hdlsllib/Logic and Bit Operations/Bit Slice  lidx=127  ridx=112
      settings: SourceProductBaseCode=SL
  Matrix Concatenate : Concatenate  NumInputs=8  ConcatenateDimension=2
  Vector : Outport
  wires:
  Bit Slice7/1 -> Matrix Concatenate/8
  Bit Slice6/1 -> Matrix Concatenate/7
  Bit Slice5/1 -> Matrix Concatenate/6
  Bit Slice4/1 -> Matrix Concatenate/5
  Bit Slice3/1 -> Matrix Concatenate/4
  Bit Slice2/1 -> Matrix Concatenate/3
  Bit Slice1/1 -> Matrix Concatenate/2
  Bit Slice0/1 -> Matrix Concatenate/1
  SSR/1 -> Bit Slice0/1, Bit Slice1/1, Bit Slice2/1, Bit Slice3/1, Bit Slice4/1, Bit Slice5/1, Bit Slice7/1, Bit Slice6/1
  Matrix Concatenate/1 -> Vector/1

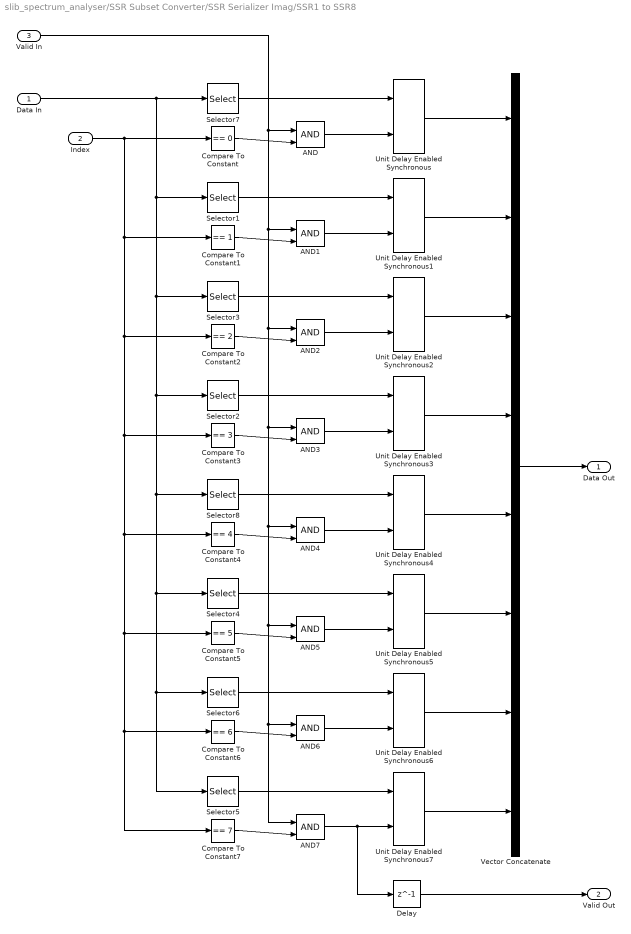
== system slib_spectrum_analyser/SSR Subset Converter/SSR Serializer Imag/SSR1 to SSR8 ==
  Data In : Inport
  Index : Inport  Port=2
  Valid In : Inport  Port=3
  AND{,1..7} (8 alike) : Logic  IconShape=distinctive  AllPortsSameDT=off  OutDataTypeStr=boolean
  Compare To Constant : simulink/Logic and Bit Operations/Compare To Constant  relop===  const=0  OutDataTypeStr=boolean
  Compare To Constant1 : simulink/Logic and Bit Operations/Compare To Constant  relop===  const=1  OutDataTypeStr=boolean
  Compare To Constant2 : simulink/Logic and Bit Operations/Compare To Constant  relop===  const=2  OutDataTypeStr=boolean
  Compare To Constant3 : simulink/Logic and Bit Operations/Compare To Constant  relop===  const=3  OutDataTypeStr=boolean
  Compare To Constant4 : simulink/Logic and Bit Operations/Compare To Constant  relop===  const=4  OutDataTypeStr=boolean
  Compare To Constant5 : simulink/Logic and Bit Operations/Compare To Constant  relop===  const=5  OutDataTypeStr=boolean
  Compare To Constant6 : simulink/Logic and Bit Operations/Compare To Constant  relop===  const=6  OutDataTypeStr=boolean
  Compare To Constant7 : simulink/Logic and Bit Operations/Compare To Constant  relop===  const=7  OutDataTypeStr=boolean
  Delay : Delay  DelayLength=1
  Selector{1..8} (8 alike) : Selector  IndexMode=Zero-based  InputPortWidth=8  IndexOptions=Index vector (dialog)  Indices=0  OutputSizes=1
  Unit Delay Enabled Synchronous{,1..7} (8 alike) : hdlsllib/Discrete/Unit Delay Enabled Synchronous  InitialCondition=0.0  SampleTime=-1
      settings: SourceProductBaseCode=SL
  Vector Concatenate : Concatenate  NumInputs=8
  Data Out : Outport
  Valid Out : Outport  Port=2
  wires:
  Unit Delay Enabled Synchronous/1 -> Vector Concatenate/1
  Unit Delay Enabled Synchronous1/1 -> Vector Concatenate/2
  Unit Delay Enabled Synchronous2/1 -> Vector Concatenate/3
  Unit Delay Enabled Synchronous3/1 -> Vector Concatenate/4
  Unit Delay Enabled Synchronous4/1 -> Vector Concatenate/5
  Unit Delay Enabled Synchronous5/1 -> Vector Concatenate/6
  Unit Delay Enabled Synchronous6/1 -> Vector Concatenate/7
  Unit Delay Enabled Synchronous7/1 -> Vector Concatenate/8
  Delay/1 -> Valid Out/1
  Vector Concatenate/1 -> Data Out/1
  Selector4/1 -> Unit Delay Enabled Synchronous5/1
  Selector8/1 -> Unit Delay Enabled Synchronous4/1
  Index/1 -> Compare To Constant/1, Compare To Constant1/1, Compare To Constant2/1, Compare To Constant3/1, Compare To Constant4/1, Compare To Constant5/1, Compare To Constant6/1, Compare To Constant7/1
  Selector5/1 -> Unit Delay Enabled Synchronous7/1
  Selector1/1 -> Unit Delay Enabled Synchronous1/1
  Selector7/1 -> Unit Delay Enabled Synchronous/1
  Selector2/1 -> Unit Delay Enabled Synchronous3/1
  Data In/1 -> Selector7/1, Selector1/1, Selector3/1, Selector2/1, Selector8/1, Selector4/1, Selector6/1, Selector5/1
  Selector6/1 -> Unit Delay Enabled Synchronous6/1
  Selector3/1 -> Unit Delay Enabled Synchronous2/1
  AND/1 -> Unit Delay Enabled Synchronous/2
  Compare To Constant/1 -> AND/2
  Valid In/1 -> AND7/1, AND6/1, AND5/1, AND4/1, AND3/1, AND2/1, AND1/1, AND/1
  AND1/1 -> Unit Delay Enabled Synchronous1/2
  AND2/1 -> Unit Delay Enabled Synchronous2/2
  AND3/1 -> Unit Delay Enabled Synchronous3/2
  AND4/1 -> Unit Delay Enabled Synchronous4/2
  AND5/1 -> Unit Delay Enabled Synchronous5/2
  AND6/1 -> Unit Delay Enabled Synchronous6/2
  AND7/1 -> Unit Delay Enabled Synchronous7/2, Delay/1
  Compare To Constant7/1 -> AND7/2
  Compare To Constant6/1 -> AND6/2
  Compare To Constant5/1 -> AND5/2
  Compare To Constant4/1 -> AND4/2
  Compare To Constant3/1 -> AND3/2
  Compare To Constant2/1 -> AND2/2
  Compare To Constant1/1 -> AND1/2

== system slib_spectrum_analyser/SSR Subset Converter/SSR Serializer Imag/SSR2 to SSR8 ==
  Data In : Inport
  Index : Inport  Port=2
  Valid In : Inport  Port=3
  AND{,1..3} (4 alike) : Logic  IconShape=distinctive  AllPortsSameDT=off  OutDataTypeStr=boolean
  Compare To Constant10 : simulink/Logic and Bit Operations/Compare To Constant  relop===  const=2  OutDataTypeStr=boolean
  Compare To Constant11 : simulink/Logic and Bit Operations/Compare To Constant  relop===  const=3  OutDataTypeStr=boolean
  Compare To Constant8 : simulink/Logic and Bit Operations/Compare To Constant  relop===  const=0  OutDataTypeStr=boolean
  Compare To Constant9 : simulink/Logic and Bit Operations/Compare To Constant  relop===  const=1  OutDataTypeStr=boolean
  Delay : Delay  DelayLength=1
  Selector{9..12} (4 alike) : Selector  IndexMode=Zero-based  InputPortWidth=8  IndexOptions=Index vector (dialog)  Indices=[0, 1]  OutputSizes=1
  Unit Delay Enabled Synchronous{,1..3} (4 alike) : hdlsllib/Discrete/Unit Delay Enabled Synchronous  InitialCondition=0.0  SampleTime=-1
      settings: SourceProductBaseCode=SL
  Vector Concatenate : Concatenate  NumInputs=4
  Data Out : Outport
  Valid Out : Outport  Port=2
  wires:
  Unit Delay Enabled Synchronous3/1 -> Vector Concatenate/4
  Unit Delay Enabled Synchronous2/1 -> Vector Concatenate/3
  Unit Delay Enabled Synchronous1/1 -> Vector Concatenate/2
  Unit Delay Enabled Synchronous/1 -> Vector Concatenate/1
  Delay/1 -> Valid Out/1
  Selector11/1 -> Unit Delay Enabled Synchronous3/1
  Selector12/1 -> Unit Delay Enabled Synchronous/1
  Index/1 -> Compare To Constant8/1, Compare To Constant9/1, Compare To Constant10/1, Compare To Constant11/1
  Vector Concatenate/1 -> Data Out/1
  Selector9/1 -> Unit Delay Enabled Synchronous1/1
  Data In/1 -> Selector12/1, Selector11/1, Selector10/1, Selector9/1
  Selector10/1 -> Unit Delay Enabled Synchronous2/1
  AND/1 -> Unit Delay Enabled Synchronous/2
  AND3/1 -> Unit Delay Enabled Synchronous3/2, Delay/1
  AND2/1 -> Unit Delay Enabled Synchronous2/2
  AND1/1 -> Unit Delay Enabled Synchronous1/2
  Compare To Constant9/1 -> AND1/2
  Compare To Constant8/1 -> AND/2
  Valid In/1 -> AND3/1, AND2/1, AND1/1, AND/1
  Compare To Constant10/1 -> AND2/2
  Compare To Constant11/1 -> AND3/2

== system slib_spectrum_analyser/SSR Subset Converter/SSR Serializer Imag/SSR4 to SSR8 ==
  Data In : Inport
  Index : Inport  Port=2
  Valid In : Inport  Port=3
  AND : Logic  IconShape=distinctive  AllPortsSameDT=off  OutDataTypeStr=boolean
  AND1 : Logic  IconShape=distinctive  AllPortsSameDT=off  OutDataTypeStr=boolean
  Compare To Constant12 : simulink/Logic and Bit Operations/Compare To Constant  relop===  const=0  OutDataTypeStr=boolean
  Compare To Constant13 : simulink/Logic and Bit Operations/Compare To Constant  relop===  const=1  OutDataTypeStr=boolean
  Delay : Delay  DelayLength=1
  Selector13 : Selector  IndexMode=Zero-based  InputPortWidth=8  IndexOptions=Index vector (dialog)  Indices=[0, 1, 2, 3]  OutputSizes=1
  Selector14 : Selector  IndexMode=Zero-based  InputPortWidth=8  IndexOptions=Index vector (dialog)  Indices=[0, 1, 2, 3]  OutputSizes=1
  Unit Delay Enabled Synchronous : hdlsllib/Discrete/Unit Delay Enabled Synchronous  InitialCondition=0.0  SampleTime=-1
      settings: SourceProductBaseCode=SL
  Unit Delay Enabled Synchronous1 : hdlsllib/Discrete/Unit Delay Enabled Synchronous  InitialCondition=0.0  SampleTime=-1
      settings: SourceProductBaseCode=SL
  Vector Concatenate : Concatenate
  Data Out : Outport
  Valid Out : Outport  Port=2
  wires:
  Delay/1 -> Valid Out/1
  Unit Delay Enabled Synchronous1/1 -> Vector Concatenate/2
  Unit Delay Enabled Synchronous/1 -> Vector Concatenate/1
  Vector Concatenate/1 -> Data Out/1
  Data In/1 -> Selector14/1, Selector13/1
  Selector13/1 -> Unit Delay Enabled Synchronous/1
  Selector14/1 -> Unit Delay Enabled Synchronous1/1
  Index/1 -> Compare To Constant13/1, Compare To Constant12/1
  AND/1 -> Unit Delay Enabled Synchronous/2
  Compare To Constant12/1 -> AND/2
  Valid In/1 -> AND1/1, AND/1
  AND1/1 -> Unit Delay Enabled Synchronous1/2, Delay/1
  Compare To Constant13/1 -> AND1/2
